simulink model "test_vehicle_model"  (R2016b)
settings: Solver=VariableStepAuto  StartTime=0.0  StopTime=10.0  RelTol=1e-3
values from neighbouring files (symbols this model uses):
  encoder_convert = 1    [test_vehicle_model.m]
  encoder_ratio = 1    [test_vehicle_model.m]
  error_convert = 1    [test_vehicle_model.m]
  gear_ratio = 1    [test_vehicle_model.m]
  k_motor = 1    [test_vehicle_model.m]
  t_motor = 1    [test_vehicle_model.m]
libraries: simulink x2
settings Model: Creator=jbarr  LastModifiedBy=jbarr

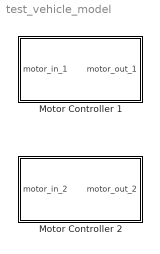
== system test_vehicle_model ==
  Motor Controller 1 : Subsystem
  Motor Controller 2 : Subsystem

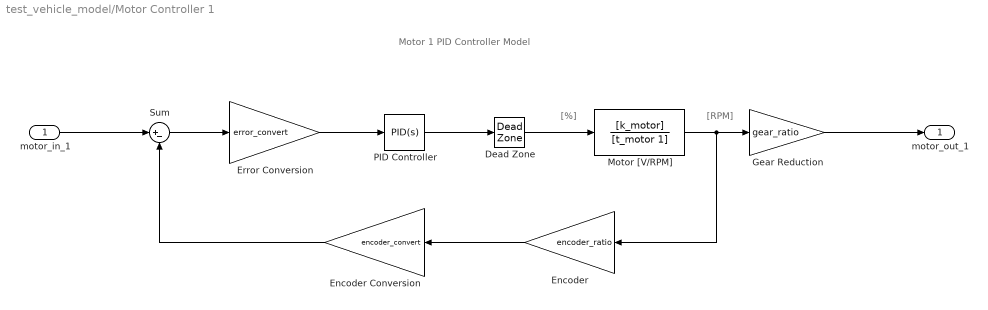
== system test_vehicle_model/Motor Controller 1 ==
  note: Motor 1 PID Controller Model
  note: [%]
  note: [RPM]
  motor_in_1 : Inport
  Dead Zone : DeadZone  SaturateOnIntegerOverflow=on
  "Encoder " : Gain  Gain=encoder_ratio
  Encoder Conversion : Gain  Gain=encoder_convert
  "Error Conversion " : Gain  Gain=error_convert
  Gear Reduction : Gain  Gain=gear_ratio
  "Motor [V/RPM] " : TransferFcn  Numerator=[k_motor]  Denominator=[t_motor 1]
  PID Controller : simulink/Continuous/PID Controller  Controller=PID  TimeDomain=Continuous-time  SampleTime=-1  IntegratorMethod=Forward Euler  FilterMethod=Forward Euler  Form=Parallel  UseFilter=on  ControllerParametersSource=internal  P=1  I=1  D=0  N=100  InitialConditionSource=internal  InitialConditionForIntegrator=0  InitialConditionForFilter=0  ExternalReset=none  LimitOutput=off  UpperSaturationLimit=inf  LowerSaturationLimit=-inf  LinearizeAsGain=on  AntiWindupMode=none  Kb=1  TrackingMode=off  Kt=1  PParamMin=[]  PParamMax=[]  IParamMin=[]  IParamMax=[]  DParamMin=[]  DParamMax=[]  NParamMin=[]  NParamMax=[]  KbParamMin=[]  KbParamMax=[]  KtParamMin=[]  KtParamMax=[]  POutMin=[]  POutMax=[]  IOutMin=[]  IOutMax=[]  DOutMin=[]  DOutMax=[]  NOutMin=[]  NOutMax=[]  KbOutMin=[]  KbOutMax=[]  KtOutMin=[]  KtOutMax=[]  IntegratorOutMin=[]  IntegratorOutMax=[]  FilterOutMin=[]  FilterOutMax=[]  SumOutMin=[]  SumOutMax=[]  SumI1OutMin=[]  SumI1OutMax=[]  SumI2OutMin=[]  SumI2OutMax=[]  SumI3OutMin=[]  SumI3OutMax=[]  SumDOutMin=[]  SumDOutMax=[]  SaturationOutMin=[]  SaturationOutMax=[]  IntegratorContinuousStateAttributes=''  IntegratorStateMustResolveToSignalObject=off  IntegratorRTWStateStorageClass=Auto  FilterContinuousStateAttributes=''  FilterStateMustResolveToSignalObject=off  FilterRTWStateStorageClass=Auto  DifferentiatorICPrevScaledInput=0  DifferentiatorOutMin=[]  DifferentiatorOutMax=[]
  Sum : Sum  Inputs=|+-
  motor_out_1 : Outport
  wires:
  Dead Zone/1 -> "Motor [V/RPM] "/1
  "Motor [V/RPM] "/1 -> "Encoder "/1, Gear Reduction/1
  "Encoder "/1 -> Encoder Conversion/1
  Sum/1 -> "Error Conversion "/1
  Encoder Conversion/1 -> Sum/2
  "Error Conversion "/1 -> PID Controller/1
  PID Controller/1 -> Dead Zone/1
  motor_in_1/1 -> Sum/1
  Gear Reduction/1 -> motor_out_1/1

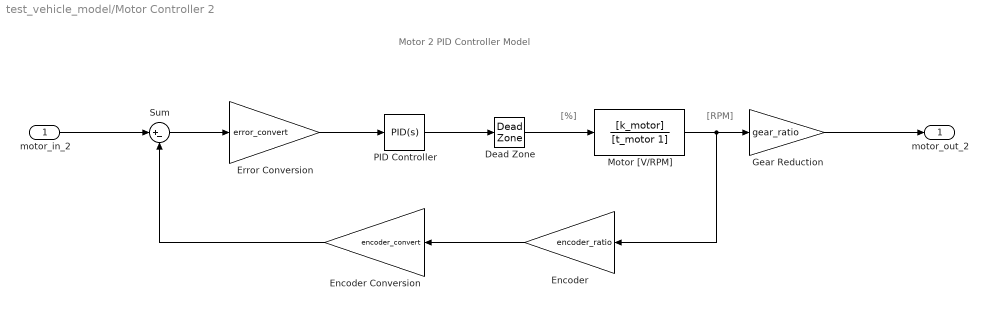
== system test_vehicle_model/Motor Controller 2 ==
  note: [RPM]
  note: [%]
  note: Motor 2 PID Controller Model
  motor_in_2 : Inport
  Dead Zone : DeadZone  SaturateOnIntegerOverflow=on
  "Encoder " : Gain  Gain=encoder_ratio
  Encoder Conversion : Gain  Gain=encoder_convert
  "Error Conversion " : Gain  Gain=error_convert
  Gear Reduction : Gain  Gain=gear_ratio
  "Motor [V/RPM] " : TransferFcn  Numerator=[k_motor]  Denominator=[t_motor 1]
  PID Controller : simulink/Continuous/PID Controller  Controller=PID  TimeDomain=Continuous-time  SampleTime=-1  IntegratorMethod=Forward Euler  FilterMethod=Forward Euler  Form=Parallel  UseFilter=on  ControllerParametersSource=internal  P=1  I=1  D=0  N=100  InitialConditionSource=internal  InitialConditionForIntegrator=0  InitialConditionForFilter=0  ExternalReset=none  LimitOutput=off  UpperSaturationLimit=inf  LowerSaturationLimit=-inf  LinearizeAsGain=on  AntiWindupMode=none  Kb=1  TrackingMode=off  Kt=1  PParamMin=[]  PParamMax=[]  IParamMin=[]  IParamMax=[]  DParamMin=[]  DParamMax=[]  NParamMin=[]  NParamMax=[]  KbParamMin=[]  KbParamMax=[]  KtParamMin=[]  KtParamMax=[]  POutMin=[]  POutMax=[]  IOutMin=[]  IOutMax=[]  DOutMin=[]  DOutMax=[]  NOutMin=[]  NOutMax=[]  KbOutMin=[]  KbOutMax=[]  KtOutMin=[]  KtOutMax=[]  IntegratorOutMin=[]  IntegratorOutMax=[]  FilterOutMin=[]  FilterOutMax=[]  SumOutMin=[]  SumOutMax=[]  SumI1OutMin=[]  SumI1OutMax=[]  SumI2OutMin=[]  SumI2OutMax=[]  SumI3OutMin=[]  SumI3OutMax=[]  SumDOutMin=[]  SumDOutMax=[]  SaturationOutMin=[]  SaturationOutMax=[]  IntegratorContinuousStateAttributes=''  IntegratorStateMustResolveToSignalObject=off  IntegratorRTWStateStorageClass=Auto  FilterContinuousStateAttributes=''  FilterStateMustResolveToSignalObject=off  FilterRTWStateStorageClass=Auto  DifferentiatorICPrevScaledInput=0  DifferentiatorOutMin=[]  DifferentiatorOutMax=[]
  Sum : Sum  Inputs=|+-
  motor_out_2 : Outport
  wires:
  Gear Reduction/1 -> motor_out_2/1
  motor_in_2/1 -> Sum/1
  PID Controller/1 -> Dead Zone/1
  "Error Conversion "/1 -> PID Controller/1
  Encoder Conversion/1 -> Sum/2
  Sum/1 -> "Error Conversion "/1
  "Encoder "/1 -> Encoder Conversion/1
  "Motor [V/RPM] "/1 -> Gear Reduction/1, "Encoder "/1
  Dead Zone/1 -> "Motor [V/RPM] "/1
